simulink model "Motor_model"  (R2025b)
settings: Solver=VariableStepAuto  StartTime=0.0  StopTime=27  RelTol=1e-3
values from neighbouring files (symbols this model uses):
  Km = 11.8676/ 12.6778    (= 0.936093012983)    [untitled.m]
  Time_const = 1 / 12.6778    (= 0.0788780387764)    [untitled.m]
settings Model: Creator=GILBERT  LastModifiedBy=GILBERT

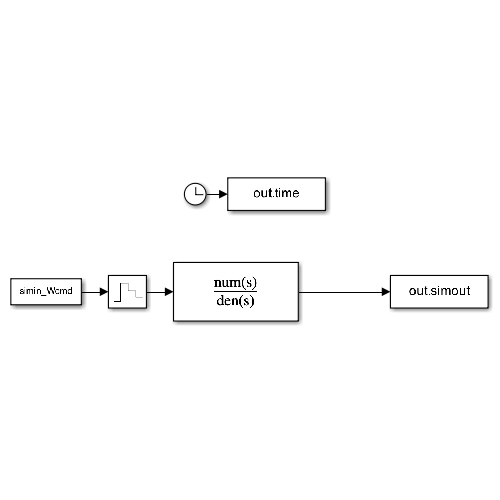
[thumbnail: Simulink's stored preview of the top-level diagram]
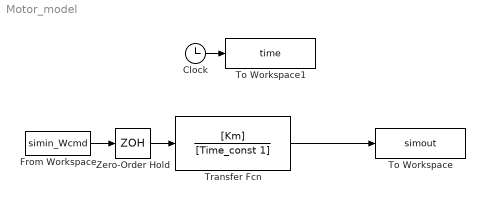
== system Motor_model ==
  Clock : Clock
  From Workspace : FromWorkspace  VariableName=simin_Wcmd
  To Workspace : ToWorkspace  VariableName=simout  SampleTime=-1
  To Workspace1 : ToWorkspace  VariableName=time  SampleTime=-1
  Transfer Fcn : TransferFcn  Numerator=[Km]  Denominator=[Time_const 1]
  Zero-Order Hold : ZeroOrderHold  SampleTime=0.05
  wires:
  Transfer Fcn/1 -> To Workspace/1
  Clock/1 -> To Workspace1/1
  From Workspace/1 -> Zero-Order Hold/1
  Zero-Order Hold/1 -> Transfer Fcn/1
